simulink model "fb_inverter1"  (Simulink 6.1)
settings: Solver=ode23tb  StartTime=0.0  StopTime=0.1499  MaxStep=5e-5  RelTol=1e-3  AbsTol=.01
libraries: powerlib x7
settings Model: LastModifiedBy=ThinkPad
settings DebuggingCC: SolverPrmCheckMsg=warning

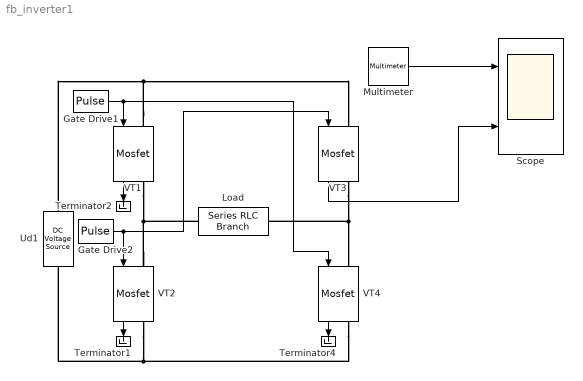
== system fb_inverter1 ==
  Gate Drive1 : DiscretePulseGenerator  PulseType=Time based  Period=0.02  PulseWidth=49.5  PhaseDelay=0.01
  Gate Drive2 : DiscretePulseGenerator  PulseType=Time based  Period=0.02  PulseWidth=49.5
  Load : powerlib/Elements/Series RLC Branch  Orientation=left  PhysicalDomain=powersysdomain  SubClassName=unknown  LeftPortType=p1  RightPortType=p1  LConnTagsString=__new0  RConnTagsString=__new0  Resistance=1  Inductance=0.01  Capacitance=inf  Measurements=Branch voltage and current
  Multimeter : powerlib/Measurements/Multimeter  PhasorSimulation=off  OutputType=Complex  sel=[1 2]  L=2  Gain=[1 1]  yselected={'Ub: Load','Ib: Load'};  PSBOutputType=1  PSBequivalent=0  AxesSetting=[0,0.1,-100,100]  Display=0  SavedBlockNames=-11
  Scope : Scope  NumInputPorts=2
      settings: TimeRange=0.05  YMin=-200~-200  YMax=200~200  SampleTime=2e-4
  Terminator1 : Terminator
      settings: Orientation=down
  Terminator2 : Terminator
      settings: Orientation=down
  Terminator4 : Terminator
      settings: Orientation=down
  Ud1 : powerlib/Electrical Sources/DC Voltage Source  Orientation=up  Amplitude=100  Measurements=None
  VT{1..4} (4 alike) : powerlib/Power Electronics/Mosfet  Orientation=down  Ron=0.01  Lon=1e-7  Rd=.01  IC=0  Rs=5  Cs=1e-6  Measurements=on
  wires:
  Gate Drive1/1 -> VT4/1, VT1/1
  Gate Drive2/1 -> VT2/1, VT3/1
  VT3/1 -> Scope/2
  Multimeter/1 -> Scope/1
  VT1/1 -> Terminator2/1
  VT2/1 -> Terminator1/1
  VT4/1 -> Terminator4/1
  connections:
  VT3/RConn1 -- VT4/LConn1 -- Load/LConn1
  VT2/LConn1 -- Load/RConn1 -- VT1/RConn1
  VT4/RConn1 -- Ud1/LConn1 -- VT2/RConn1
  VT1/LConn1 -- VT3/LConn1 -- Ud1/RConn1
